simulink model "vehicle_model"  (R2024b)
settings: Solver=VariableStepAuto  StartTime=0.0  StopTime=10.0  RelTol=1e-3
values from neighbouring files (symbols this model uses):
  PAR_BODY_v_InitVelocity = Simulink.Parameter    [vehicle_body_params.m]
libraries: nesl_utility x15, sdl_lib x9, fl_lib x2
settings Model: Creator=rocke  LastModifiedBy=rocke

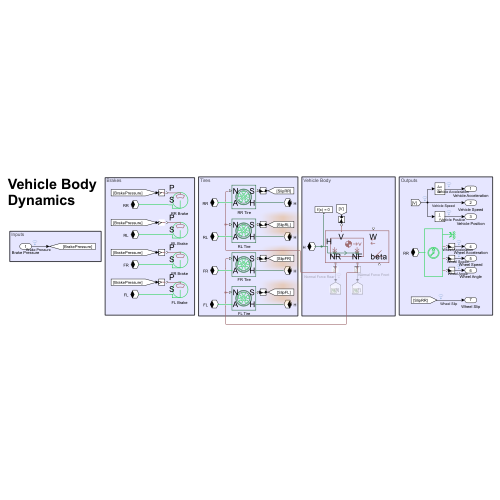
[thumbnail: Simulink's stored preview of the top-level diagram]
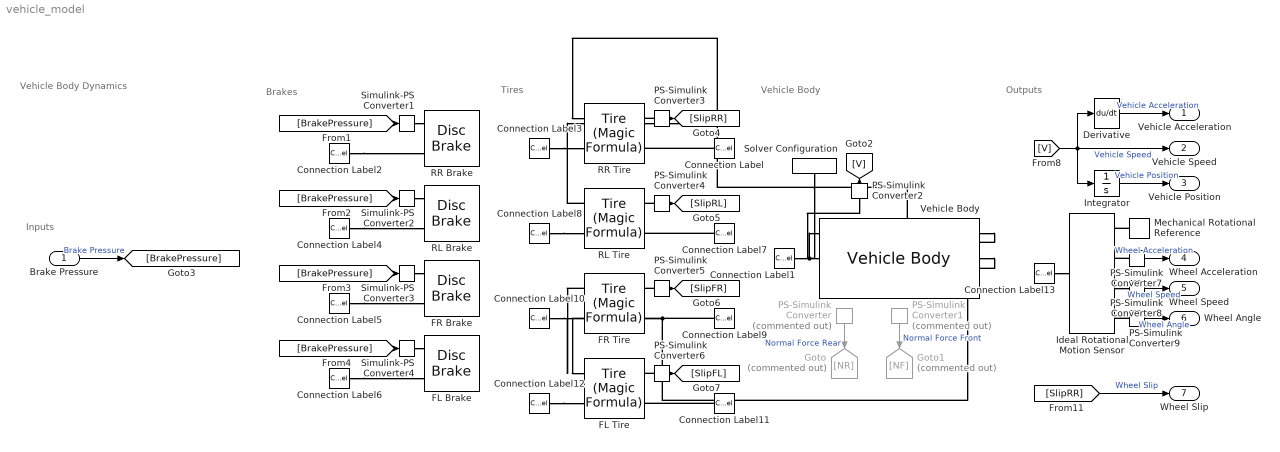
== system vehicle_model ==
  note: Vehicle Body
      | Dynamics
  note: Outputs
  note: Tires
  note: Vehicle Body
  note: Inputs
  note: Brakes
  Brake Pressure : Inport
  Connection Label{,1,7,9,11} (5 alike) : ConnectionLabel  Label=H
  Connection Label10 : ConnectionLabel  Label=FR
  Connection Label12 : ConnectionLabel  Label=FL
  Connection Label13 : ConnectionLabel  Label=RR
  Connection Label2 : ConnectionLabel  Label=RR
  Connection Label3 : ConnectionLabel  Label=RR
  Connection Label4 : ConnectionLabel  Label=RL
  Connection Label5 : ConnectionLabel  Label=FR
  Connection Label6 : ConnectionLabel  Label=FL
  Connection Label8 : ConnectionLabel  Label=RL
  Derivative : Derivative
  FL Brake : sdl_lib/Brakes & Detents/Rotational/Disc Brake  r_mean=150 mm  bore=10 mm  n_pads=2  thermal_port=simscape.enum.thermaleffects.omit  mu_static=0.9  mu_coulomb=0.7  temperature_TLU=[280, 300, 320] K  mu_static_TLU=[.9, .8, .7]  mu_coulomb_TLU=[.8, .7, .6]  brkwy_vel=0.1 rad/s  visc_coef=0 N*m*s/rad  thermal_mass=50 kJ/K  temperature_specify=off  temperature_priority=High  temperature=300 K  temperature_nominal_specify=off  temperature_nominal_value=1  temperature_nominal_unit=K
  FL Tire : sdl_lib/Tires & Vehicles/Tire (Magic Formula)  parameterization=sdl.enum.magic_tire_model.peak  F_z1=PAR_TIRE_f_RatedVerLoad N  F_x1=PAR_TIRE_f_PeakLongForce N  kappa1=PAR_TIRE_nr_SlipAtPeakForce  B_m=10  C_m=1.9  D_m=1  E_m=0.97  fz0=4000 N  p_Cx=1.685  p_Dx=[1.21, -.037]  p_Ex=[.344, .095, -.02, 0]  p_Kx=[21.51, -.163, .245]  p_Hx=[-.002, .002]  p_Vx=[0, 0]  rolling_radius_model=sdl.enum.RollingRadiusParameterization.Constant  r_e=PAR_TIRE_d_RollingRadius m  r_0=0.3 m  breff=8.39  dreff=0.26  freff=0.074  q_re0=0.99  q_v1=0.008  longvl=17 m/s  cz=5e5 N/m  model_resistance=false  resistance_model=sdl.enum.rollingResistanceParameterization.constant  coeff=0.015  p_tire=250e3 Pa  alpha=-0.003  beta=0.97  coeff_a=84e-4  coeff_b=6.2e-4 s/m  coeff_c=1.6e-4 s^2/m^2  p_tire0=240e3 Pa  fz0_resistance=4000 N  vH0=16 m/s  q_Sy=[.0082, 0, .0014, .001, 0, 0, 1.08, -.5]  v_thr=0.001 m/s  enable_scaling_coefficients=false  lfzO=1  lcx=1  lmux=1  lex=1  lkx=1  lhx=1  lvx=1  lmy=1  model_compliance=sdl.enum.compliance.off  stiffness=1e6 N/m  damping=1000 N*s/m  model_inertia=sdl.enum.model_inertia.on  inertia=PAR_TIRE_j_Inertia kg*m^2  initial_velocity=PAR_TIRE_agv_InitSpeed rad/s  vxlow=1 m/s  v_tr_thr=0.1 m/s  kpumin=-1.5  kpumax=1.5
  FR Brake : sdl_lib/Brakes & Detents/Rotational/Disc Brake  r_mean=150 mm  bore=10 mm  n_pads=2  thermal_port=simscape.enum.thermaleffects.omit  mu_static=0.9  mu_coulomb=0.7  temperature_TLU=[280, 300, 320] K  mu_static_TLU=[.9, .8, .7]  mu_coulomb_TLU=[.8, .7, .6]  brkwy_vel=0.1 rad/s  visc_coef=0 N*m*s/rad  thermal_mass=50 kJ/K  temperature_specify=off  temperature_priority=High  temperature=300 K  temperature_nominal_specify=off  temperature_nominal_value=1  temperature_nominal_unit=K
  FR Tire : sdl_lib/Tires & Vehicles/Tire (Magic Formula)  parameterization=sdl.enum.magic_tire_model.peak  F_z1=PAR_TIRE_f_RatedVerLoad N  F_x1=PAR_TIRE_f_PeakLongForce N  kappa1=PAR_TIRE_nr_SlipAtPeakForce  B_m=10  C_m=1.9  D_m=1  E_m=0.97  fz0=4000 N  p_Cx=1.685  p_Dx=[1.21, -.037]  p_Ex=[.344, .095, -.02, 0]  p_Kx=[21.51, -.163, .245]  p_Hx=[-.002, .002]  p_Vx=[0, 0]  rolling_radius_model=sdl.enum.RollingRadiusParameterization.Constant  r_e=PAR_TIRE_d_RollingRadius m  r_0=0.3 m  breff=8.39  dreff=0.26  freff=0.074  q_re0=0.99  q_v1=0.008  longvl=17 m/s  cz=5e5 N/m  model_resistance=false  resistance_model=sdl.enum.rollingResistanceParameterization.constant  coeff=0.015  p_tire=250e3 Pa  alpha=-0.003  beta=0.97  coeff_a=84e-4  coeff_b=6.2e-4 s/m  coeff_c=1.6e-4 s^2/m^2  p_tire0=240e3 Pa  fz0_resistance=4000 N  vH0=16 m/s  q_Sy=[.0082, 0, .0014, .001, 0, 0, 1.08, -.5]  v_thr=0.001 m/s  enable_scaling_coefficients=false  lfzO=1  lcx=1  lmux=1  lex=1  lkx=1  lhx=1  lvx=1  lmy=1  model_compliance=sdl.enum.compliance.off  stiffness=1e6 N/m  damping=1000 N*s/m  model_inertia=sdl.enum.model_inertia.on  inertia=PAR_TIRE_j_Inertia kg*m^2  initial_velocity=PAR_TIRE_agv_InitSpeed rad/s  vxlow=1 m/s  v_tr_thr=0.1 m/s  kpumin=-1.5  kpumax=1.5
  Goto : Goto  Commented=on  GotoTag=NR
  Goto1 : Goto  Commented=on  GotoTag=NF
  Ideal Rotational Motion Sensor : fl_lib/Mechanical/Mechanical Sensors/Ideal Rotational Motion Sensor  reference=foundation.enum.MeasurementReference.difference  acceleration_port=true  velocity_port=true  position_port=true  wrap_angle=false  offset=0 rad
      settings: InternalSimscapePortConfiguration="{\"Bottom\":[],\"Left\":[{\"id\":\"R\",\"label\":\"R\",\"type\":\"foundation.mechanical.rotational.rotational\"}],\"Right\":[{\"id\":\"C\",\"label\":\"C\",\"type\":\"foundation.mechanical.rotational.rotational\"},{\"id\":\"alpha\",\"label\":\"α\",\"type\":\"output\"},{\"id\":\"W\",\"label\":\"W\",\"type\":\"output\"},{\"id\":\"A\",\"label\":\"A\",\"type\":\"output\"}],\"Top\":[]}"
  Integrator : Integrator
  Mechanical Rotational Reference : fl_lib/Mechanical/Rotational Elements/Mechanical Rotational Reference
  PS-Simulink Converter : nesl_utility/PS-Simulink Converter  Commented=on  PhysicalDomain=network_engine_domain  SubClassName=ps_output  LeftPortType=input  RightPortType=output  PseudoPeriodic=off  Frequencies=[]  VectorFormat=inherit  Unit=inherit  AffineConversion=off
  PS-Simulink Converter1 : nesl_utility/PS-Simulink Converter  Commented=on  PhysicalDomain=network_engine_domain  SubClassName=ps_output  LeftPortType=input  RightPortType=output  PseudoPeriodic=off  Frequencies=[]  VectorFormat=inherit  Unit=inherit  AffineConversion=off
  PS-Simulink Converter{2..9} (8 alike) : nesl_utility/PS-Simulink Converter  PhysicalDomain=network_engine_domain  SubClassName=ps_output  LeftPortType=input  RightPortType=output  PseudoPeriodic=off  Frequencies=[]  VectorFormat=inherit  Unit=inherit  AffineConversion=off
  RL Brake : sdl_lib/Brakes & Detents/Rotational/Disc Brake  r_mean=150 mm  bore=10 mm  n_pads=2  thermal_port=simscape.enum.thermaleffects.omit  mu_static=0.9  mu_coulomb=0.7  temperature_TLU=[280, 300, 320] K  mu_static_TLU=[.9, .8, .7]  mu_coulomb_TLU=[.8, .7, .6]  brkwy_vel=0.1 rad/s  visc_coef=0 N*m*s/rad  thermal_mass=50 kJ/K  temperature_specify=off  temperature_priority=High  temperature=300 K  temperature_nominal_specify=off  temperature_nominal_value=1  temperature_nominal_unit=K
  RL Tire : sdl_lib/Tires & Vehicles/Tire (Magic Formula)  parameterization=sdl.enum.magic_tire_model.peak  F_z1=PAR_TIRE_f_RatedVerLoad N  F_x1=PAR_TIRE_f_PeakLongForce N  kappa1=PAR_TIRE_nr_SlipAtPeakForce  B_m=10  C_m=1.9  D_m=1  E_m=0.97  fz0=4000 N  p_Cx=1.685  p_Dx=[1.21, -.037]  p_Ex=[.344, .095, -.02, 0]  p_Kx=[21.51, -.163, .245]  p_Hx=[-.002, .002]  p_Vx=[0, 0]  rolling_radius_model=sdl.enum.RollingRadiusParameterization.Constant  r_e=PAR_TIRE_d_RollingRadius m  r_0=0.3 m  breff=8.39  dreff=0.26  freff=0.074  q_re0=0.99  q_v1=0.008  longvl=17 m/s  cz=5e5 N/m  model_resistance=false  resistance_model=sdl.enum.rollingResistanceParameterization.constant  coeff=0.015  p_tire=250e3 Pa  alpha=-0.003  beta=0.97  coeff_a=84e-4  coeff_b=6.2e-4 s/m  coeff_c=1.6e-4 s^2/m^2  p_tire0=240e3 Pa  fz0_resistance=4000 N  vH0=16 m/s  q_Sy=[.0082, 0, .0014, .001, 0, 0, 1.08, -.5]  v_thr=0.001 m/s  enable_scaling_coefficients=false  lfzO=1  lcx=1  lmux=1  lex=1  lkx=1  lhx=1  lvx=1  lmy=1  model_compliance=sdl.enum.compliance.off  stiffness=1e6 N/m  damping=1000 N*s/m  model_inertia=sdl.enum.model_inertia.on  inertia=PAR_TIRE_j_Inertia kg*m^2  initial_velocity=PAR_TIRE_agv_InitSpeed rad/s  vxlow=1 m/s  v_tr_thr=0.1 m/s  kpumin=-1.5  kpumax=1.5
  RR Brake : sdl_lib/Brakes & Detents/Rotational/Disc Brake  r_mean=150 mm  bore=10 mm  n_pads=2  thermal_port=simscape.enum.thermaleffects.omit  mu_static=0.9  mu_coulomb=0.7  temperature_TLU=[280, 300, 320] K  mu_static_TLU=[.9, .8, .7]  mu_coulomb_TLU=[.8, .7, .6]  brkwy_vel=0.1 rad/s  visc_coef=0 N*m*s/rad  thermal_mass=50 kJ/K  temperature_specify=off  temperature_priority=High  temperature=300 K  temperature_nominal_specify=off  temperature_nominal_value=1  temperature_nominal_unit=K
  RR Tire : sdl_lib/Tires & Vehicles/Tire (Magic Formula)  parameterization=sdl.enum.magic_tire_model.peak  F_z1=PAR_TIRE_f_RatedVerLoad N  F_x1=PAR_TIRE_f_PeakLongForce N  kappa1=PAR_TIRE_nr_SlipAtPeakForce  B_m=10  C_m=1.9  D_m=1  E_m=0.97  fz0=4000 N  p_Cx=1.685  p_Dx=[1.21, -.037]  p_Ex=[.344, .095, -.02, 0]  p_Kx=[21.51, -.163, .245]  p_Hx=[-.002, .002]  p_Vx=[0, 0]  rolling_radius_model=sdl.enum.RollingRadiusParameterization.Constant  r_e=PAR_TIRE_d_RollingRadius m  r_0=0.3 m  breff=8.39  dreff=0.26  freff=0.074  q_re0=0.99  q_v1=0.008  longvl=17 m/s  cz=5e5 N/m  model_resistance=false  resistance_model=sdl.enum.rollingResistanceParameterization.constant  coeff=0.015  p_tire=250e3 Pa  alpha=-0.003  beta=0.97  coeff_a=84e-4  coeff_b=6.2e-4 s/m  coeff_c=1.6e-4 s^2/m^2  p_tire0=240e3 Pa  fz0_resistance=4000 N  vH0=16 m/s  q_Sy=[.0082, 0, .0014, .001, 0, 0, 1.08, -.5]  v_thr=0.001 m/s  enable_scaling_coefficients=false  lfzO=1  lcx=1  lmux=1  lex=1  lkx=1  lhx=1  lvx=1  lmy=1  model_compliance=sdl.enum.compliance.off  stiffness=1e6 N/m  damping=1000 N*s/m  model_inertia=sdl.enum.model_inertia.on  inertia=PAR_TIRE_j_Inertia kg*m^2  initial_velocity=PAR_TIRE_agv_InitSpeed rad/s  vxlow=1 m/s  v_tr_thr=0.1 m/s  kpumin=-1.5  kpumax=1.5
  Simulink-PS Converter{1..4} (4 alike) : nesl_utility/Simulink-PS Converter  PhysicalDomain=network_engine_domain  SubClassName=ps_input  LeftPortType=input  RightPortType=output  PseudoPeriodic=off  Frequencies=[]  NoiseDistribution=none  NoiseParameters=[]  Unit=1  AffineConversion=off  FilteringAndDerivatives=provide  SimscapeFilterOrder=1  InputFilterTimeConstant=0.001  UdotUserProvided=0
  Solver Configuration : nesl_utility/Solver Configuration  PhysicalDomain=network_engine_domain  SubClassName=solver  LeftPortType=input  RightPortType=generic  Tones=[]  Harmonics=[]  SimulateNoise=off  Profile=off  UseLocalSampling=off  EnableSwitchedLinearOptims=on  FrequencyDomain=off  UseCCode=off  RelTol=0.001  AbsTol=0.001  MinStep=1e-09  ToWorkspace=off  RevertToSquareIcSolve=off  NumHomotopyIterations=100  PhasorMode=off  PhasorModeNumHarmonics=1  ConsistencySolver=NEWTON_XTOL_AFTER_FTOL  IndexReductionMethod=DerivativeReplacement  DoDC=off  ResidualTolerance=1e-09  ConsistencyTolSource=GLOBAL  ConsistencyAbsTol=0.001  ConsistencyRelTol=0.001  ConsistencyTolFactor=0.001  UseLocalSolver=off  LocalSolverChoice=NE_BACKWARD_EULER_ADVANCER  ResolveIndetEquations=on  FunctionEvalNumThread=1  LocalSolverSampleTime=0.001  DoFixedCost=off  MaxNonlinIter=3  MaxModeIter=2  ComputeImpulses=off  ImpulseIterations=2  LinearAlgebra=auto  LinearAlgebraNumThread=0  EquationFormulation=NE_TIME_EF  DelaysMemoryBudget=1024  AutomaticFiltering=on  FilteringTimeConstant=0.001  PartitionStorageMethod=AS_NEEDED  PartitionMemoryBudget=1024  PartitionMethod=ROBUST  MultibodyUseLocalSolver=off  MultibodyLocalSolverChoice=ODE1  MultibodyLocalSolverSampleTime=0.001
  Vehicle Body : sdl_lib/Tires & Vehicles/Vehicle Body  mass=PAR_BODY_m_Mass kg  n_w=PAR_BODY_nr_Wheels  x_f=PAR_BODY_d_FrontToCG m  x_r=PAR_BODY_d_RearToCG m  y_c=PAR_BODY_d_HeightCG m  mass_var=false  g=9.81 m/s^2  liftoff_warning=false  area=PAR_BODY_a_FrontalArea m^2  Cd_var=false  Cd=PAR_BODY_nr_DragCoeff  rho=PAR_BODY_rho_AirDensity kg/m^3  model_pitch=false  inertia=4000 kg*m^2  suspension_model=sdl.enum.linearTLU.linear  k_f=1e4 N/m  b_f=1e4 N*s/m  k_r=1e4 N/m  b_r=1e4 N*s/m  k_f_TLU=[-2000, -1000, 0, 1000, 2000] N  x_f_TLU=[-.4, -.2, 0, .2, .4] m  b_f_TLU=[-200, -100, 0, 100, 200] N  v_f_TLU=[-4, -2, 0, 2, 4] m/s  k_r_TLU=[-2000, -1000, 0, 1000, 2000] N  x_r_TLU=[-.4, -.2, 0, .2, .4] m  b_r_TLU=[-200, -100, 0, 100, 200] N  v_r_TLU=[-4, -2, 0, 2, 4] m/s  interp_method=simscape.enum.interpolation.linear  extrap_method=simscape.enum.extrapolation.linear  model_hardstop=false  upper_bound_f=.25 m  lower_bound_f=-.25 m  stop_k_f=1e6 N/m  stop_b_f=150 N*s/m  upper_bound_r=.25 m  lower_bound_r=-.25 m  stop_k_r=1e6 N/m  stop_b_r=150 N*s/m  initial_pitch=0 rad  initial_pitch_rate=0 rad/s  v_specify=on  v_priority=High  v=PAR_BODY_v_InitVelocity/3.6 m/s  v_nominal_specify=off  v_nominal_value=1  v_nominal_unit=m/s
      settings: InternalSimscapePortConfiguration="{\"Bottom\":[{\"id\":\"NR\",\"label\":\"NR\",\"type\":\"output\"},{\"id\":\"NF\",\"label\":\"NF\",\"type\":\"output\"},{\"id\":\"beta\",\"label\":\"beta\",\"type\":\"input\"}],\"Left\":[{\"id\":\"H\",\"label\":\"H\",\"type\":\"foundation.mechanical.translational.translational\"}],\"Right\":[],\"Top\":[{\"id\":\"V\",\"label\":\"V\",\"type\":\"output\"},{\"id\":\"wind\",\"label\":\"W\",\"type\":\"input\"}]}"
  Vehicle Acceleration : Outport
  Vehicle Speed : Outport  Port=2
  Vehicle Position : Outport  Port=3
  Wheel Acceleration : Outport  Port=4
  Wheel Speed : Outport  Port=5
  Wheel Angle : Outport  Port=6
  Wheel Slip : Outport  Port=7
  wires:
  PS-Simulink Converter/1 -> Goto/1  "Normal Force Rear"
  PS-Simulink Converter1/1 -> Goto1/1  "Normal Force Front"
  Brake Pressure/1 -> [BrakePressure]  "Brake Pressure"
  [BrakePressure] -> Simulink-PS Converter1/1
  [BrakePressure] -> Simulink-PS Converter2/1
  [BrakePressure] -> Simulink-PS Converter3/1
  [BrakePressure] -> Simulink-PS Converter4/1
  PS-Simulink Converter3/1 -> [SlipRR]
  PS-Simulink Converter4/1 -> [SlipRL]
  PS-Simulink Converter5/1 -> [SlipFR]
  PS-Simulink Converter6/1 -> [SlipFL]
  PS-Simulink Converter2/1 -> [V]
  PS-Simulink Converter7/1 -> Wheel Acceleration/1  "Wheel Acceleration"
  PS-Simulink Converter9/1 -> Wheel Angle/1  "Wheel Angle"
  PS-Simulink Converter8/1 -> Wheel Speed/1  "Wheel Speed"
  [V] -> Integrator/1, Vehicle Speed/1, Derivative/1  "Vehicle Speed"
  Derivative/1 -> Vehicle Acceleration/1  "Vehicle Acceleration"
  Integrator/1 -> Vehicle Position/1  "Vehicle Position"
  [SlipRR] -> Wheel Slip/1  "Wheel Slip"
  connections:
  PS-Simulink Converter2/LConn1 -- Vehicle Body/LConn2
  Vehicle Body/RConn1 -- RL Tire/LConn1 -- RR Tire/LConn1
  Connection Label/LConn1 -- RR Tire/RConn2
  Connection Label1/LConn1 -- Vehicle Body/LConn1 -- Solver Configuration/RConn1
  Connection Label2/LConn1 -- RR Brake/LConn2
  Connection Label3/LConn1 -- RR Tire/LConn2
  Simulink-PS Converter1/RConn1 -- RR Brake/LConn1
  Simulink-PS Converter2/RConn1 -- RL Brake/LConn1
  Connection Label4/LConn1 -- RL Brake/LConn2
  Simulink-PS Converter3/RConn1 -- FR Brake/LConn1
  Connection Label5/LConn1 -- FR Brake/LConn2
  Simulink-PS Converter4/RConn1 -- FL Brake/LConn1
  Connection Label6/LConn1 -- FL Brake/LConn2
  PS-Simulink Converter3/LConn1 -- RR Tire/RConn1
  PS-Simulink Converter4/LConn1 -- RL Tire/RConn1
  Connection Label8/LConn1 -- RL Tire/LConn2
  Connection Label7/LConn1 -- RL Tire/RConn2
  Connection Label10/LConn1 -- FR Tire/LConn2
  Connection Label11/LConn1 -- FL Tire/RConn2
  Connection Label12/LConn1 -- FL Tire/LConn2
  Connection Label9/LConn1 -- FR Tire/RConn2
  PS-Simulink Converter6/LConn1 -- FL Tire/RConn1
  Vehicle Body/RConn2 -- FR Tire/LConn1 -- FL Tire/LConn1
  PS-Simulink Converter5/LConn1 -- FR Tire/RConn1
  Connection Label13/LConn1 -- Ideal Rotational Motion Sensor/LConn1
  Mechanical Rotational Reference/LConn1 -- Ideal Rotational Motion Sensor/RConn1
  PS-Simulink Converter7/LConn1 -- Ideal Rotational Motion Sensor/RConn2
  PS-Simulink Converter9/LConn1 -- Ideal Rotational Motion Sensor/RConn4
  Ideal Rotational Motion Sensor/RConn3 -- PS-Simulink Converter8/LConn1
